simulink model "pdControl_unittest"  (R2018b)
settings: Solver=VariableStepAuto  StartTime=0.0  StopTime=100  RelTol=1e-3
values from neighbouring files (symbols this model uses):
  quat_cmd = quat_cmd/norm(quat_cmd)    [pdController_unittest_init.m]
  w_cmd_radps = zeros(3,1)    [pdController_unittest_init.m]
undefined symbols (not defined in the file or in its folder): simParams
libraries: PD_Controller_Lib x1, quat_err_lib x1, quat_kinematics_lib x1, rigid_body_dynamics_lib x1
settings Model: Creator=colem  LastModifiedBy=Taylor

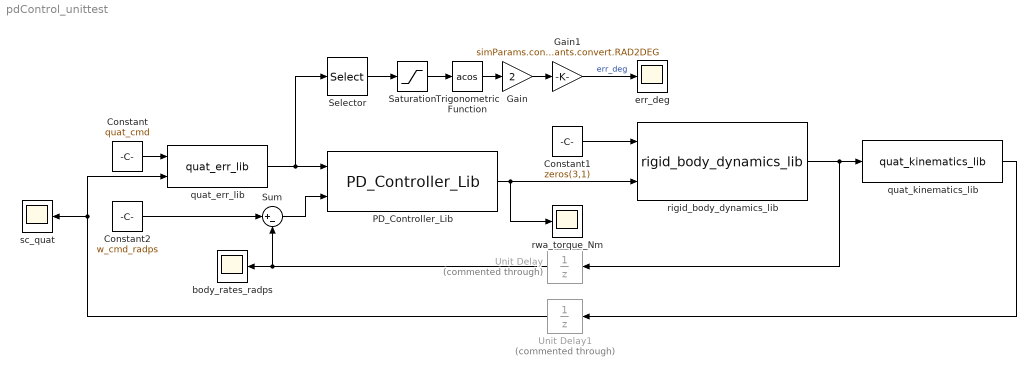
== system pdControl_unittest ==
  Constant : Constant  Value=quat_cmd
  Constant1 : Constant  Value=zeros(3,1)
  Constant2 : Constant  Value=w_cmd_radps
  Gain : Gain  Gain=2
  Gain1 : Gain  Gain=simParams.constants.convert.RAD2DEG
  PD_Controller_Lib : PD_Controller_Lib/PD_Controller_Lib  SystemSampleTime=-1
  Saturation : Saturate  UpperLimit=1  LowerLimit=-1
  Selector : Selector  InputPortWidth=4  IndexOptions=Index vector (dialog)  Indices=[1]  OutputSizes=1
  Sum : Sum  Inputs=|+-
  Trigonometric Function : Trigonometry  Operator=acos
  Unit Delay : UnitDelay  Commented=through  InitialCondition=simParams.initialConditions.w_body_radps  SampleTime=-1
  Unit Delay1 : UnitDelay  Commented=through  InitialCondition=simParams.initialConditions.q_eci2body  SampleTime=-1
  body_rates_radps : Scope
  err_deg : Scope
  quat_err_lib : quat_err_lib/quat_err_lib  SystemSampleTime=-1
  quat_kinematics_lib : quat_kinematics_lib/quat_kinematics_lib  SystemSampleTime=-1
  rigid_body_dynamics_lib : rigid_body_dynamics_lib/rigid_body_dynamics_lib  SystemSampleTime=-1
  rwa_torque_Nm : Scope
  sc_quat : Scope
  wires:
  quat_err_lib/1 -> Selector/1, PD_Controller_Lib/1
  Constant1/1 -> rigid_body_dynamics_lib/1
  Trigonometric Function/1 -> Gain/1
  quat_kinematics_lib/1 -> Unit Delay1/1
  rigid_body_dynamics_lib/1 -> Unit Delay/1, quat_kinematics_lib/1
  Unit Delay/1 -> Sum/2, body_rates_radps/1
  Unit Delay1/1 -> sc_quat/1, quat_err_lib/2
  Saturation/1 -> Trigonometric Function/1
  Selector/1 -> Saturation/1
  Gain/1 -> Gain1/1
  Gain1/1 -> err_deg/1  "err_deg"
  Sum/1 -> PD_Controller_Lib/2
  Constant/1 -> quat_err_lib/1
  Constant2/1 -> Sum/1
  PD_Controller_Lib/1 -> rigid_body_dynamics_lib/2, rwa_torque_Nm/1
